simulink model "det_thd_tb"  (R2014a)
settings: Solver=FixedStepDiscrete  StartTime=0.0  StopTime=64  FixedStep=1  RelTol=1e-3
libraries: simulink x2, hdlsllib x1
settings Model: Creator=User  LastModifiedBy=User

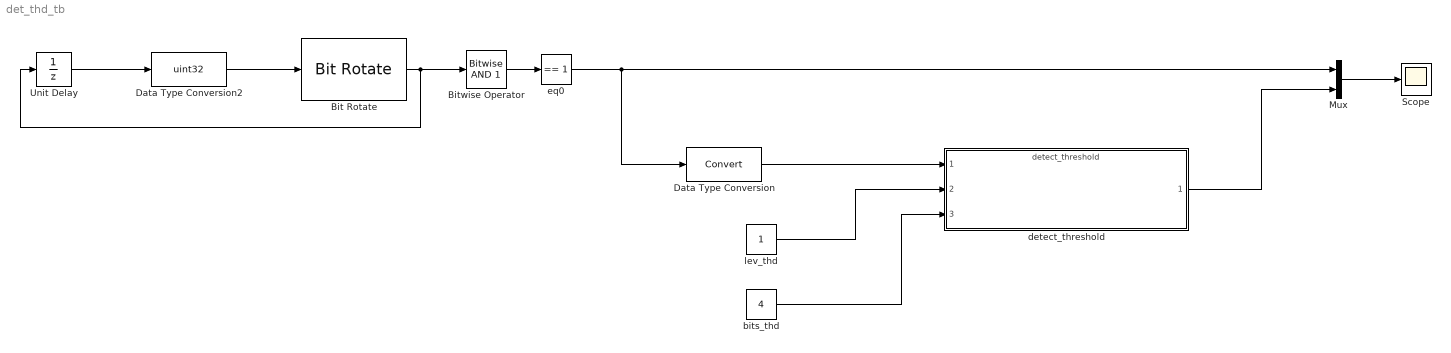
== system det_thd_tb ==
  Bit Rotate : hdlsllib/HDL Operations/Bit Rotate  mode=Rotate Left  N=1
  Bitwise Operator : simulink/Logic and Bit Operations/Bitwise Operator  logicop=AND  UseBitMask=on  BitMask=1  BitMaskRealWorld=Stored Integer
  Data Type Conversion : DataTypeConversion
  Data Type Conversion2 : DataTypeConversion  OutDataTypeStr=uint32
  Mux : Mux  Inputs=2
  Scope : Scope
      settings: MaxDataPoints=500000
  Unit Delay : UnitDelay  InitialCondition=bin2dec('00001110000000000001111000000000')  SampleTime=-1
  bits_thd : Constant  Value=4  OutDataTypeStr=fixdt(1,16,0)
  detect_threshold : ModelReference  ModelNameDialog=detect_threshold.slx  SimulationMode=Normal  ModelReferenceVersion=1.39  CopyOfModelName=detect_threshold.slx  DefaultDataLogging=on
  eq0 : simulink/Logic and Bit Operations/Compare To Constant  relop===  const=1  OutDataTypeStr=boolean
  lev_thd : Constant  OutDataTypeStr=fixdt(1,16,0)
  wires:
  Unit Delay/1 -> Data Type Conversion2/1
  Bit Rotate/1 -> Bitwise Operator/1, Unit Delay/1
  Bitwise Operator/1 -> eq0/1
  eq0/1 -> Mux/1, Data Type Conversion/1
  Data Type Conversion/1 -> detect_threshold/1
  lev_thd/1 -> detect_threshold/2
  Data Type Conversion2/1 -> Bit Rotate/1
  Mux/1 -> Scope/1
  detect_threshold/1 -> Mux/2
  bits_thd/1 -> detect_threshold/3
